simulink model "tst"  (R2023a)
settings: Solver=VariableStepAuto  StartTime=0.0  StopTime=10.0  RelTol=1e-3
values from neighbouring files (symbols this model uses):
  D = 0:0.01:0.9    [limit_cycle_est.m]
undefined symbols (not defined in the file or in its folder): aMode
libraries: simulink_extras x3, shared6dofsys x1, sharedutil x1
settings Model: Creator=s3928  LastModifiedBy=cnsl

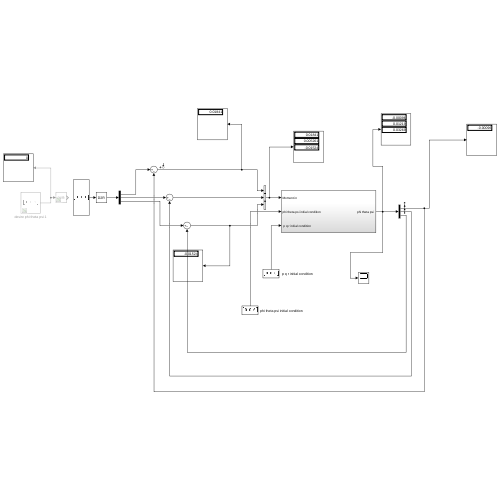
[thumbnail: Simulink's stored preview of the top-level diagram]
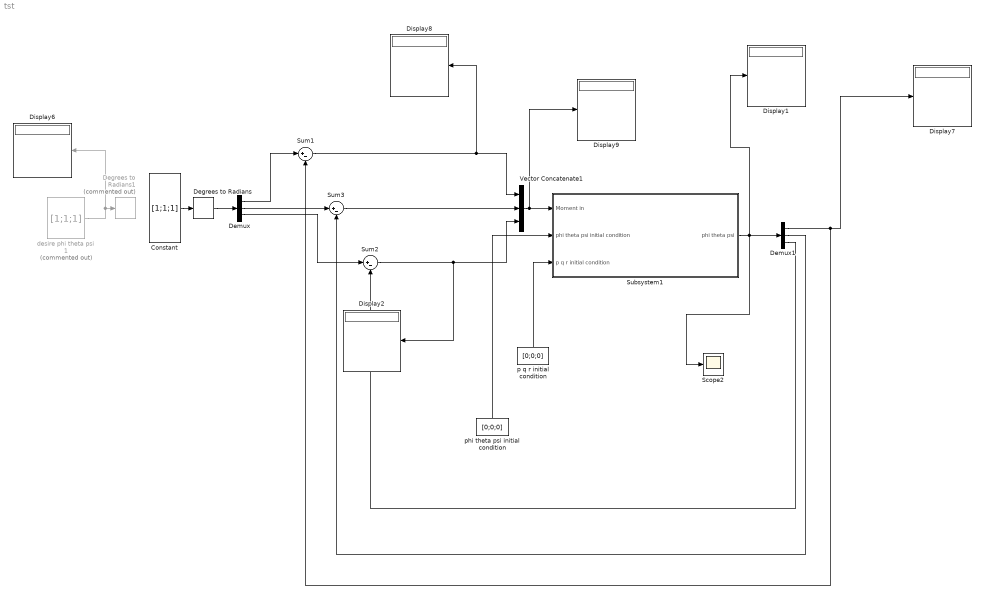
== system tst ==
  " p q r initial condition" : Constant  Value=[0;0;0]
  Constant : Constant  Value=[1;1;1]
  Degrees to Radians : simulink_extras/Transformations/Degrees to Radians
  Degrees to Radians1 : simulink_extras/Transformations/Degrees to Radians  Commented=on
  Demux : Demux  Outputs=3
  Demux1 : Demux  Outputs=3
  Display{1..2,6..9} (6 alike) : Display
  Scope2 : Scope
  Subsystem1 : Subsystem
  Sum1 : Sum  Inputs=|+-
  Sum2 : Sum  Inputs=|+-
  Sum3 : Sum  Inputs=|+-
  Vector Concatenate1 : Concatenate  NumInputs=3
  desire phi theta psi 1 : Constant  Commented=on  Value=[1;1;1]
  "phi theta psi initial condition " : Constant  Value=[0;0;0]
  wires:
  Demux1/1 -> Display7/1, Sum1/2
  Subsystem1/1("phi theta psi ") -> Display1/1, Demux1/1, Scope2/1
  Sum3/1 -> Vector Concatenate1/2
  desire phi theta psi 1/1 -> Display6/1, Degrees to Radians1/1
  "phi theta psi initial condition "/1 -> Subsystem1/2("phi theta psi initial condition ")
  Sum1/1 -> Vector Concatenate1/1, Display8/1
  Vector Concatenate1/1 -> Display9/1, Subsystem1/1(Moment in)
  " p q r initial condition"/1 -> Subsystem1/3(" p q r initial condition")
  Demux/1 -> Sum1/1
  Demux/2 -> Sum3/1
  Demux/3 -> Sum2/1
  Sum2/1 -> Display2/1, Vector Concatenate1/3
  Constant/1 -> Degrees to Radians/1
  Degrees to Radians/1 -> Demux/1
  Demux1/2 -> Sum3/2
  Demux1/3 -> Sum2/2

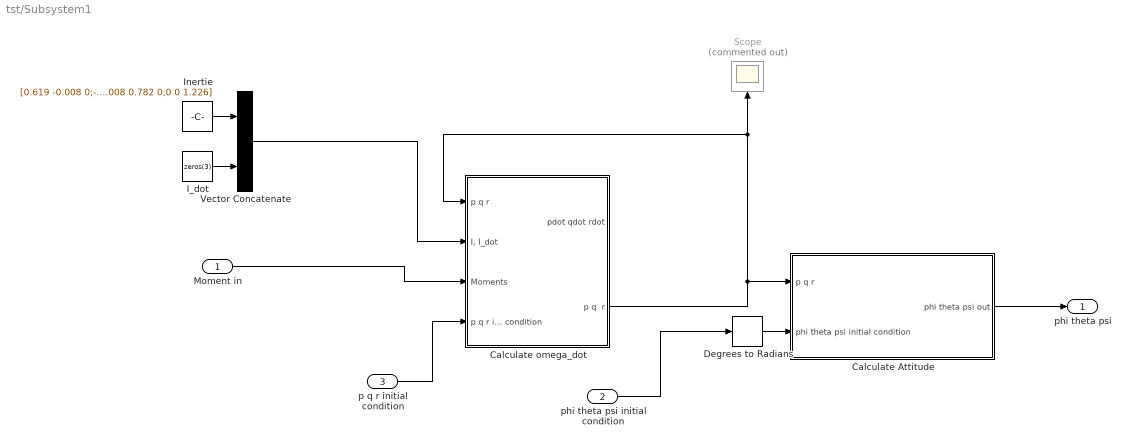
== system tst/Subsystem1 ==
  Moment in : Inport
  "phi theta psi initial condition " : Inport  Port=2
  " p q r initial condition" : Inport  Port=3
  "Calculate Attitude " : Subsystem
  Calculate omega_dot : Subsystem  AncestorBlock=shared6dofsys/Calculate omega_dot  mask{aMode=aMode}
      mask init:
      | if aerosharedtest(gcb)
      |     aerosharedicon('shared');
      | else
      |     sharedautoicon('shared');
      | end
      settings: LibrarySourceBlock=shared6dofsys/Calculate omega_dot
  Degrees to Radians : simulink_extras/Transformations/Degrees to Radians
  I_dot : Constant  Value=zeros(3)
  Inertie : Constant  Value=[0.619 -0.008 0;-0.008 0.782 0;0 0 1.226]
  Scope : Scope  Commented=on
  Vector Concatenate : Concatenate  Mode=Multidimensional array
  "phi theta psi " : Outport
  wires:
  Vector Concatenate/1 -> Calculate omega_dot/2("I, I_dot")
  Inertie/1 -> Vector Concatenate/1
  Calculate omega_dot/2(p q  r) -> Scope/1, Calculate omega_dot/1(p q r), "Calculate Attitude "/1(p q r)
  I_dot/1 -> Vector Concatenate/2
  Moment in/1 -> Calculate omega_dot/3(Moments)
  "Calculate Attitude "/1("phi theta psi out ") -> "phi theta psi "/1
  Degrees to Radians/1 -> "Calculate Attitude "/2("phi theta psi initial condition ")
  "phi theta psi initial condition "/1 -> Degrees to Radians/1
  " p q r initial condition"/1 -> Calculate omega_dot/4(p q r initial condition)

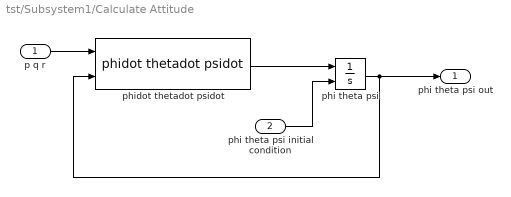
== system tst/Subsystem1/Calculate Attitude  ==
  p q r : Inport
  "phi theta psi initial condition " : Inport  Port=2
  " phi theta psi" : Integrator  InitialConditionSource=external
  phidot thetadot psidot : shared6dofsys/DCM & Euler Angles (Euler)/phidot thetadot psidot  SystemSampleTime=-1  VariantActivationTime=update diagram  Latency=0  AutoFrameSizeCalculation=off
  "phi theta psi out " : Outport
  wires:
  "phi theta psi initial condition "/1 -> " phi theta psi"/2
  " phi theta psi"/1 -> phidot thetadot psidot/2, "phi theta psi out "/1
  phidot thetadot psidot/1 -> " phi theta psi"/1
  p q r/1 -> phidot thetadot psidot/1

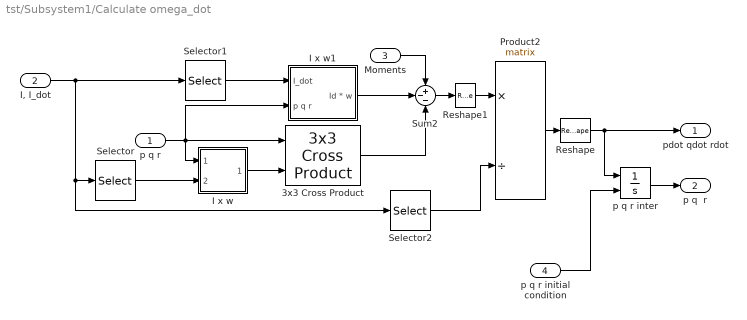
== system tst/Subsystem1/Calculate omega_dot ==
  p q r : Inport  OutDataTypeStr=double
  "I, I_dot" : Inport  Port=2  OutDataTypeStr=double
  Moments : Inport  Port=3  OutDataTypeStr=double
  p q r initial condition : Inport  Port=4
  3x3 Cross Product : sharedutil/3x3 Cross Product  aMode=aMode
  I x w : Subsystem
  I x w1 : Subsystem
  Product2 : Product  Inputs=*/  Multiplication=Matrix(*)  SaturateOnIntegerOverflow=on  OutDataTypeStr=Inherit: Same as first input
  Reshape : Reshape
  Reshape1 : Reshape  OutputDimensionality=Row vector (2-D)
  Selector : Selector  NumberOfDimensions=2  InputPortWidth=2  IndexOptions=Index vector (dialog),Select all  Indices=1:3,-1  OutputSizes=1
  Selector1 : Selector  NumberOfDimensions=2  InputPortWidth=2  IndexOptions=Index vector (dialog),Select all  Indices=4:6,-1  OutputSizes=1
  Selector2 : Selector  NumberOfDimensions=2  InputPortWidth=2  IndexOptions=Index vector (dialog),Select all  Indices=1:3,-1  OutputSizes=1
  Sum2 : Sum  Inputs=+--  SaturateOnIntegerOverflow=on
  p q r inter : Integrator  InitialConditionSource=external
  pdot qdot rdot : Outport  OutDataTypeStr=double  VectorParamsAs1DForOutWhenUnconnected=off
  p q  r : Outport  Port=2
  wires:
  p q r initial condition/1 -> p q r inter/2
  p q r inter/1 -> p q  r/1
  Reshape/1 -> pdot qdot rdot/1, p q r inter/1
  Selector/1 -> I x w/2(Inertia)
  Selector2/1 -> Product2/2
  "I, I_dot"/1 -> Selector/1, Selector2/1, Selector1/1
  p q r/1 -> 3x3 Cross Product/1, I x w1/2(p q r), I x w/1(p q r)
  Product2/1 -> Reshape/1
  Sum2/1 -> Reshape1/1
  Moments/1 -> Sum2/1
  I x w1/1(Id * w) -> Sum2/2
  Selector1/1 -> I x w1/1(I_dot)
  3x3 Cross Product/1 -> Sum2/3
  I x w/1(I * w) -> 3x3 Cross Product/2
  Reshape1/1 -> Product2/1

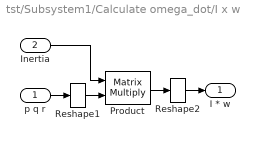
== system tst/Subsystem1/Calculate omega_dot/I x w ==
  p q r : Inport
  Inertia : Inport  Port=2
  Product : Product  Multiplication=Matrix(*)  InputSameDT=on  SaturateOnIntegerOverflow=on  OutDataTypeStr=Inherit: Same as first input
  Reshape1 : Reshape  OutputDimensionality=Column vector (2-D)
  Reshape2 : Reshape
  I * w : Outport  VectorParamsAs1DForOutWhenUnconnected=off
  wires:
  Product/1 -> Reshape2/1
  Inertia/1 -> Product/1
  p q r/1 -> Reshape1/1
  Reshape1/1 -> Product/2
  Reshape2/1 -> I * w/1

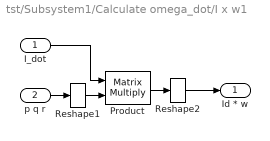
== system tst/Subsystem1/Calculate omega_dot/I x w1 ==
  I_dot : Inport
  p q r : Inport  Port=2
  Product : Product  Multiplication=Matrix(*)  InputSameDT=on  SaturateOnIntegerOverflow=on  OutDataTypeStr=Inherit: Same as first input
  Reshape1 : Reshape  OutputDimensionality=Column vector (2-D)
  Reshape2 : Reshape
  Id * w : Outport  VectorParamsAs1DForOutWhenUnconnected=off
  wires:
  p q r/1 -> Reshape1/1
  I_dot/1 -> Product/1
  Product/1 -> Reshape2/1
  Reshape1/1 -> Product/2
  Reshape2/1 -> Id * w/1
